simulink subsystem "CasADi"  (R2024b)
settings: Solver=VariableStepAuto  StartTime=0.0  StopTime=10.0  RelTol=1e-3
settings Model: Creator=thatf  LastModifiedBy=thatf

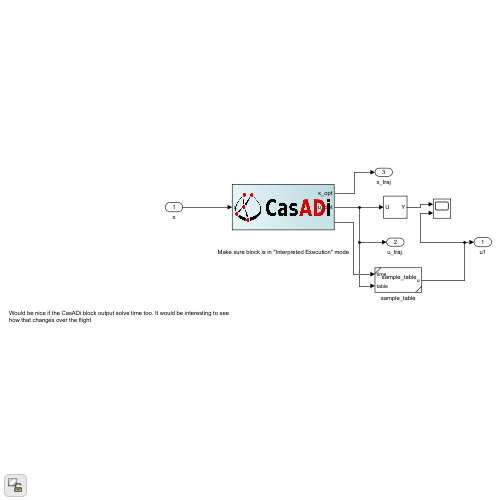
[thumbnail: Simulink's stored preview of the top-level diagram]
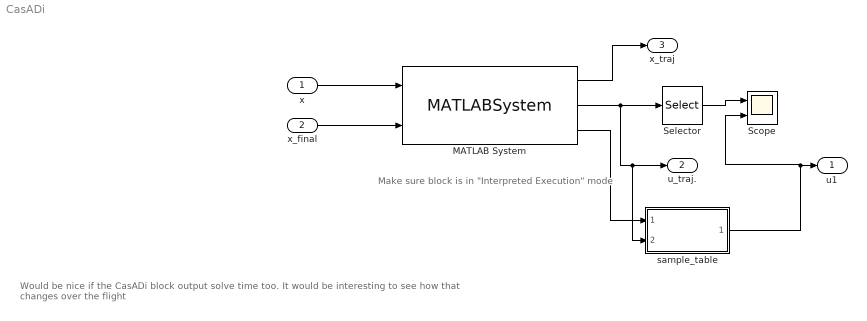
== system CasADi ==
  note: Make sure block is in "Interpreted Execution" mode
  note: Would be nice if the CasADi block output solve time too. It would be interesting to see how that changes over the flight
  x : Inport
  x_final : Inport  Port=2
  MATLAB System : MATLABSystem  System=CasADi_MPC  vehicle=vehicle  t_step=dtime  steps=steps  max_iter=max_iter  x_initial=x0  SimulateUsing=Interpreted execution  x_final=xf
      mask Type: CasADi_MPC
      mask Display:
      | image('CasADi.png');
      | port_label('input',1,'x');
      | port_label('input',2,'x_final');
      | port_label('output',1,'x_opt');
      | port_label('output',2,'u_opt');
      | port_label('output',3,'tf_opt');
  Scope : Scope  NumInputPorts=2
  Selector : Selector  NumberOfDimensions=2  InputPortWidth=3  IndexOptions=Index vector (dialog),Select all  Indices=[1],1  OutputSizes=1,1
  sample_table : Subsystem  ReferencedSubsystem=sample_table
  u1 : Outport
  u_traj. : Outport  Port=2
  x_traj : Outport  Port=3
  wires:
  Selector/1 -> Scope/1
  x/1 -> MATLAB System/1
  MATLAB System/1 -> x_traj/1
  MATLAB System/2 -> Selector/1, u_traj./1, sample_table/2
  sample_table/1 -> u1/1, Scope/2
  MATLAB System/3 -> sample_table/1
  x_final/1 -> MATLAB System/2
